simulink model "feedback_control"  (R2019a)
settings: Solver=FixedStepDiscrete  StartTime=0.0  StopTime=10.0  FixedStep=0.01  RelTol=1e-3
undefined symbols (not defined in the file): Adt, Bdt, c, DiscIntNeverNeededParam, pid, PID_pitch, PID_roll
libraries: simulink x2
settings Model: DataDictionary=pidSMC.sldd  Creator=david  LastModifiedBy=david

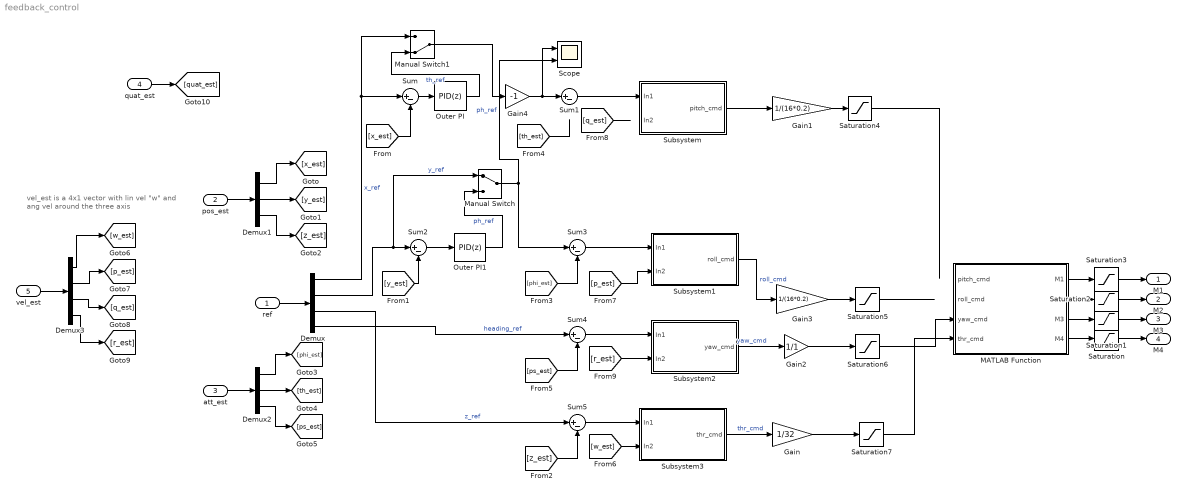
== system feedback_control ==
  note: vel_est is a 4x1 vector with lin vel "w" and
      | ang vel around the three axis
  ref : Inport
  pos_est : Inport  Port=2
  att_est : Inport  Port=3
  quat_est : Inport  Port=4
  vel_est : Inport  Port=5
  Demux : Demux
  Demux1 : Demux  Outputs=3
  Demux2 : Demux  Outputs=3
  Demux3 : Demux
  Gain : Gain  Gain=1/32
  Gain1 : Gain  Gain=1/(16*0.2)
  Gain2 : Gain  Gain=1/1
  Gain3 : Gain  Gain=1/(16*0.2)
  Gain4 : Gain  Gain=-1
  MATLAB Function : MATLAB Function  TreatAsAtomicUnit=on
  Manual Switch : ManualSwitch
  Manual Switch1 : ManualSwitch  CurrentSetting=0
  Outer PI : simulink/Continuous/PID Controller  Controller=PID  Form=Parallel  TimeDomain=Discrete-time  SampleTime=-1  IntegratorMethod=Forward Euler  FilterMethod=Forward Euler  ControllerParametersSource=internal  P=PID_pitch.Kp_out  I=PID_pitch.Ki_out  D=PID_pitch.Kd_out  UseFilter=off  N=pid.N  TunerSelectOption=Transfer Function Based (PID Tuner App)  InitialConditionSource=internal  InitialConditionForIntegrator=0  InitialConditionForFilter=0  DifferentiatorICPrevScaledInput=0  ExternalReset=none  TrackingMode=off  Kt=1  LimitOutput=on  UpperSaturationLimit=30/180*pi  LowerSaturationLimit=-30/180*pi  LinearizeAsGain=off  AntiWindupMode=clamping  Kb=1  POutMin=[]  POutMax=[]  IOutMin=[]  IOutMax=[]  DOutMin=[]  DOutMax=[]  NOutMin=[]  NOutMax=[]  SumOutMin=[]  SumOutMax=[]  SaturationOutMin=[]  SaturationOutMax=[]  PParamMin=[]  PParamMax=[]  IParamMin=[]  IParamMax=[]  DParamMin=[]  DParamMax=[]  NParamMin=[]  NParamMax=[]  KbParamMin=[]  KbParamMax=[]  KtParamMin=[]  KtParamMax=[]  KbOutMin=[]  KbOutMax=[]  KtOutMin=[]  KtOutMax=[]  IntegratorOutMin=[]  IntegratorOutMax=[]  FilterOutMin=[]  FilterOutMax=[]  SumI1OutMin=[]  SumI1OutMax=[]  SumI2OutMin=[]  SumI2OutMax=[]  SumI3OutMin=[]  SumI3OutMax=[]  SumI4OutMin=[]  SumI4OutMax=[]  SumDOutMin=[]  SumDOutMax=[]  DifferentiatorOutMin=[]  DifferentiatorOutMax=[]  FilterDiffOutCoefMin=[]  FilterDiffOutCoefMax=[]  ReciprocalOutMin=[]  ReciprocalOutMax=[]  SumDenOutMin=[]  SumDenOutMax=[]  SumNumOutMin=[]  SumNumOutMax=[]  DivideOutMin=[]  DivideOutMax=[]  IntegratorContinuousStateAttributes=''  IntegratorStateMustResolveToSignalObject=off  IntegratorRTWStateStorageClass=Auto  FilterContinuousStateAttributes=''  FilterStateMustResolveToSignalObject=off  FilterRTWStateStorageClass=Auto  ParallelPVariant=InternalParameters  IdealPVariant=Disabled  IVariant=InternalParameters  DVariant=InternalParameters  IntegratorVariant=Discrete  SatVariant=Enabled  AWVariant=DiscClampingParallel  PCopyVariant=Disabled  TRVariant=Disabled  FdbkBlocksVariant=Forward  IdealPFdbkVariant=Disabled  SatFdbkVariant=Disabled  DerivativeFilterVariant=Differentiator  NVariant=Passthrough  NCopyVariant=Disabled_SignalSpec  FilterICVariant=InternalICsDifferentiator  IntegratorICVariant=InternalICs  ExternalResetVariant=Disabled  TRSumVariant=Passthrough  SumFdbkVariant=Disabled  SumVariant=Sum_PID
  Outer PI1 : simulink/Continuous/PID Controller  Controller=PID  Form=Parallel  TimeDomain=Discrete-time  SampleTime=-1  IntegratorMethod=Forward Euler  FilterMethod=Forward Euler  ControllerParametersSource=internal  P=PID_roll.Kp_out  I=PID_roll.Ki_out  D=PID_roll.Kd_out  UseFilter=off  N=pid.N  TunerSelectOption=Transfer Function Based (PID Tuner App)  InitialConditionSource=internal  InitialConditionForIntegrator=0  InitialConditionForFilter=0  DifferentiatorICPrevScaledInput=0  ExternalReset=none  TrackingMode=off  Kt=1  LimitOutput=on  UpperSaturationLimit=30/180*pi  LowerSaturationLimit=-30/180*pi  LinearizeAsGain=off  AntiWindupMode=clamping  Kb=1  POutMin=[]  POutMax=[]  IOutMin=[]  IOutMax=[]  DOutMin=[]  DOutMax=[]  NOutMin=[]  NOutMax=[]  SumOutMin=[]  SumOutMax=[]  SaturationOutMin=[]  SaturationOutMax=[]  PParamMin=[]  PParamMax=[]  IParamMin=[]  IParamMax=[]  DParamMin=[]  DParamMax=[]  NParamMin=[]  NParamMax=[]  KbParamMin=[]  KbParamMax=[]  KtParamMin=[]  KtParamMax=[]  KbOutMin=[]  KbOutMax=[]  KtOutMin=[]  KtOutMax=[]  IntegratorOutMin=[]  IntegratorOutMax=[]  FilterOutMin=[]  FilterOutMax=[]  SumI1OutMin=[]  SumI1OutMax=[]  SumI2OutMin=[]  SumI2OutMax=[]  SumI3OutMin=[]  SumI3OutMax=[]  SumI4OutMin=[]  SumI4OutMax=[]  SumDOutMin=[]  SumDOutMax=[]  DifferentiatorOutMin=[]  DifferentiatorOutMax=[]  FilterDiffOutCoefMin=[]  FilterDiffOutCoefMax=[]  ReciprocalOutMin=[]  ReciprocalOutMax=[]  SumDenOutMin=[]  SumDenOutMax=[]  SumNumOutMin=[]  SumNumOutMax=[]  DivideOutMin=[]  DivideOutMax=[]  IntegratorContinuousStateAttributes=''  IntegratorStateMustResolveToSignalObject=off  IntegratorRTWStateStorageClass=Auto  FilterContinuousStateAttributes=''  FilterStateMustResolveToSignalObject=off  FilterRTWStateStorageClass=Auto  ParallelPVariant=InternalParameters  IdealPVariant=Disabled  IVariant=InternalParameters  DVariant=InternalParameters  IntegratorVariant=Discrete  SatVariant=Enabled  AWVariant=DiscClampingParallel  PCopyVariant=Disabled  TRVariant=Disabled  FdbkBlocksVariant=Forward  IdealPFdbkVariant=Disabled  SatFdbkVariant=Disabled  DerivativeFilterVariant=Differentiator  NVariant=Passthrough  NCopyVariant=Disabled_SignalSpec  FilterICVariant=InternalICsDifferentiator  IntegratorICVariant=InternalICs  ExternalResetVariant=Disabled  TRSumVariant=Passthrough  SumFdbkVariant=Disabled  SumVariant=Sum_PID
  Saturation : Saturate  UpperLimit=2000  LowerLimit=0
  Saturation1 : Saturate  UpperLimit=2000  LowerLimit=0
  Saturation2 : Saturate  UpperLimit=2000  LowerLimit=0
  Saturation3 : Saturate  UpperLimit=2000  LowerLimit=1000
  Saturation4 : Saturate  UpperLimit=1  LowerLimit=-1
  Saturation5 : Saturate  UpperLimit=1  LowerLimit=-1
  Saturation6 : Saturate  UpperLimit=1  LowerLimit=-1
  Saturation7 : Saturate  UpperLimit=1  LowerLimit=0
  Scope : Scope  NumInputPorts=2
  Subsystem : Subsystem
  Subsystem1 : Subsystem
  Subsystem2 : Subsystem
  Subsystem3 : Subsystem
  Sum{,1..5} (6 alike) : Sum  Inputs=|+-
  M1 : Outport
  M2 : Outport  Port=2
  M3 : Outport  Port=3
  M4 : Outport  Port=4
  wires:
  Outer PI/1 -> Manual Switch1/2  "th_ref"
  [x_est] -> Sum/2
  Saturation/1 -> M4/1
  Manual Switch/1 -> Sum3/1, Scope/2  "ph_ref"
  Demux/2 -> Manual Switch/1, Sum2/1  "y_ref"
  Gain3/1 -> Saturation5/1
  Gain/1 -> Saturation7/1
  Sum3/1 -> Subsystem1/1(In1)
  Outer PI1/1 -> Manual Switch/2  "ph_ref"
  ref/1 -> Demux/1
  Saturation2/1 -> M2/1
  vel_est/1 -> Demux3/1
  Demux3/1 -> [w_est]
  Gain1/1 -> Saturation4/1
  Saturation6/1 -> MATLAB Function/3(yaw_cmd)
  Gain2/1 -> Saturation6/1
  Gain4/1 -> Scope/1, Sum1/1
  Demux3/2 -> [p_est]
  MATLAB Function/2(M2) -> Saturation2/1
  Demux2/2 -> [th_est]
  Saturation3/1 -> M1/1
  [y_est] -> Sum2/2
  Saturation1/1 -> M3/1
  Saturation5/1 -> ?
  Demux3/3 -> [q_est]
  MATLAB Function/3(M3) -> Saturation1/1
  Saturation7/1 -> MATLAB Function/4(thr_cmd)
  Demux1/3 -> [z_est]
  Demux3/4 -> [r_est]
  Demux2/1 -> [phi_est]
  pos_est/1 -> Demux1/1
  Demux2/3 -> [ps_est]
  att_est/1 -> Demux2/1
  [phi_est] -> Sum3/2
  Demux1/2 -> [y_est]
  Demux1/1 -> [x_est]
  Demux/3 -> Sum5/1  "z_ref"
  [p_est] -> Subsystem1/2(In2)
  [r_est] -> Subsystem2/2(In2)
  Sum4/1 -> Subsystem2/1(In1)
  Subsystem1/1(roll_cmd) -> Gain3/1  "roll_cmd"
  [th_est] -> ?
  Subsystem2/1(yaw_cmd) -> Gain2/1  "yaw_cmd"
  Sum2/1 -> Outer PI1/1
  [ps_est] -> Sum4/2
  Demux/4 -> Sum4/1  "heading_ref"
  Subsystem3/1(thr_cmd) -> Gain/1  "thr_cmd"
  Sum/1 -> Outer PI/1
  Demux/1 -> Manual Switch1/1, Sum/1  "x_ref"
  MATLAB Function/1(M1) -> Saturation3/1
  [w_est] -> Subsystem3/2(In2)
  Saturation4/1 -> ?
  Sum5/1 -> Subsystem3/1(In1)
  Manual Switch1/1 -> Gain4/1
  [z_est] -> Sum5/2
  MATLAB Function/4(M4) -> Saturation/1
  Sum1/1 -> Subsystem/1(In1)
  [q_est] -> ?
  Subsystem/1(pitch_cmd) -> Gain1/1
  quat_est/1 -> [quat_est]

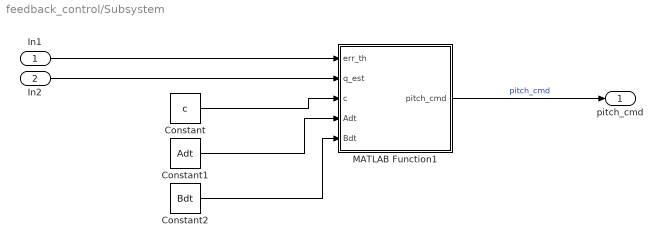
== system feedback_control/Subsystem ==
  In1 : Inport
  In2 : Inport  Port=2
  Constant : Constant  Value=c
  Constant1 : Constant  Value=Adt
  Constant2 : Constant  Value=Bdt
  MATLAB Function1 : MATLAB Function  TreatAsAtomicUnit=on
  pitch_cmd : Outport
  wires:
  MATLAB Function1/1(pitch_cmd) -> pitch_cmd/1  "pitch_cmd"
  In2/1 -> MATLAB Function1/2(q_est)
  In1/1 -> MATLAB Function1/1(err_th)
  Constant/1 -> MATLAB Function1/3(c)
  Constant1/1 -> MATLAB Function1/4(Adt)
  Constant2/1 -> MATLAB Function1/5(Bdt)

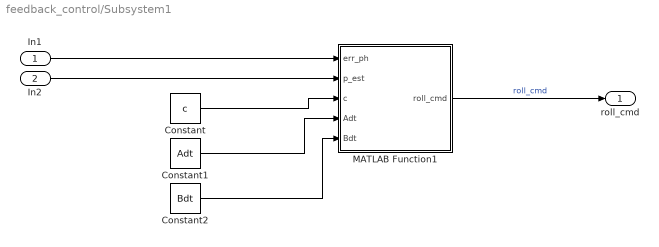
== system feedback_control/Subsystem1 ==
  In1 : Inport
  In2 : Inport  Port=2
  Constant : Constant  Value=c
  Constant1 : Constant  Value=Adt
  Constant2 : Constant  Value=Bdt
  MATLAB Function1 : MATLAB Function  TreatAsAtomicUnit=on
  roll_cmd : Outport
  wires:
  Constant2/1 -> MATLAB Function1/5(Bdt)
  Constant1/1 -> MATLAB Function1/4(Adt)
  Constant/1 -> MATLAB Function1/3(c)
  In1/1 -> MATLAB Function1/1(err_ph)
  In2/1 -> MATLAB Function1/2(p_est)
  MATLAB Function1/1(roll_cmd) -> roll_cmd/1  "roll_cmd"

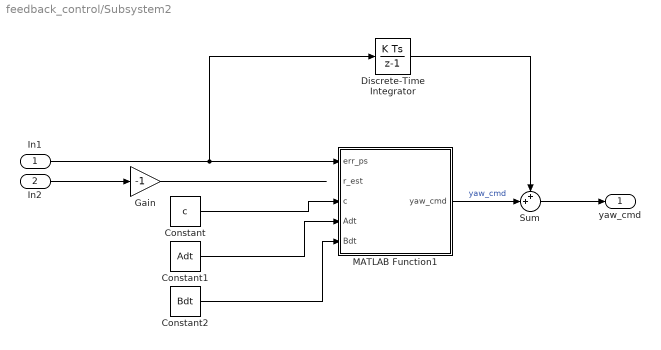
== system feedback_control/Subsystem2 ==
  In1 : Inport
  In2 : Inport  Port=2
  Constant : Constant  Value=c
  Constant1 : Constant  Value=Adt
  Constant2 : Constant  Value=Bdt
  Discrete-Time Integrator : DiscreteIntegrator  gainval=0.001  SampleTime=-1  ICPrevOutput=DiscIntNeverNeededParam  ICPrevScaledInput=DiscIntNeverNeededParam
  Gain : Gain  Gain=-1
  MATLAB Function1 : MATLAB Function  TreatAsAtomicUnit=on
  Sum : Sum  Inputs=++|
  yaw_cmd : Outport
  wires:
  MATLAB Function1/1(yaw_cmd) -> Sum/2  "yaw_cmd"
  In2/1 -> Gain/1
  In1/1 -> Discrete-Time Integrator/1, MATLAB Function1/1(err_ps)
  Constant/1 -> MATLAB Function1/3(c)
  Constant1/1 -> MATLAB Function1/4(Adt)
  Constant2/1 -> MATLAB Function1/5(Bdt)
  Sum/1 -> yaw_cmd/1
  Discrete-Time Integrator/1 -> Sum/1
  Gain/1 -> ?

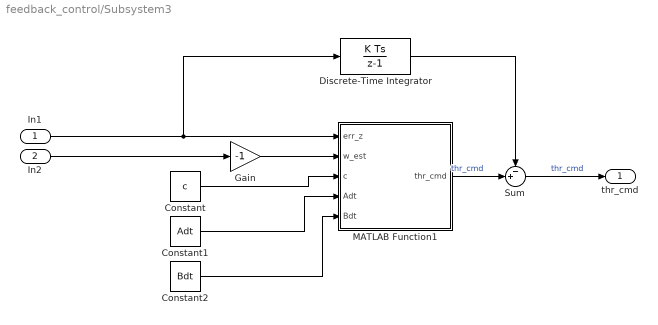
== system feedback_control/Subsystem3 ==
  In1 : Inport
  In2 : Inport  Port=2
  Constant : Constant  Value=c
  Constant1 : Constant  Value=Adt
  Constant2 : Constant  Value=Bdt
  Discrete-Time Integrator : DiscreteIntegrator  gainval=2  SampleTime=-1  LimitOutput=on  UpperSaturationLimit=20  LowerSaturationLimit=-20  ICPrevOutput=DiscIntNeverNeededParam  ICPrevScaledInput=DiscIntNeverNeededParam
  Gain : Gain  Gain=-1
  MATLAB Function1 : MATLAB Function  TreatAsAtomicUnit=on
  Sum : Sum  Inputs=-+|
  thr_cmd : Outport
  wires:
  Constant2/1 -> MATLAB Function1/5(Bdt)
  Constant1/1 -> MATLAB Function1/4(Adt)
  Constant/1 -> MATLAB Function1/3(c)
  Sum/1 -> thr_cmd/1  "thr_cmd"
  In2/1 -> Gain/1
  MATLAB Function1/1(thr_cmd) -> Sum/2  "thr_cmd"
  Discrete-Time Integrator/1 -> Sum/1
  Gain/1 -> MATLAB Function1/2(w_est)
  In1/1 -> MATLAB Function1/1(err_z), Discrete-Time Integrator/1

== matlab function feedback_control/Subsystem/MATLAB Function1 ==
  data: err_th input; pitch_cmd output; q_est input; c input; Adt input; Bdt input
function pitch_cmd = pitchSMC(err_th,q_est,c,Adt,Bdt)

pitch_cmd = inv(c'*Bdt)*c'*Adt*[ err_th; q_est ];

end

== matlab function feedback_control/MATLAB Function ==
  data: pitch_cmd input; M1 output; roll_cmd input; yaw_cmd input; thr_cmd input; M2 output; M3 output; M4 output
function [M1, M2, M3, M4] = motor_mixer(pitch_cmd, roll_cmd, yaw_cmd, thr_cmd)

idle = 1000;
K_thr = 800;
K_roll = 500;
K_pitch = 500;
K_yaw = 500;

% out = idle*ones(4,1) + K_thr*eye(4)*thr_cmd + K_roll*diag([-1, 1, 1, -1])*...
%     roll_cmd + K_pitch*diag([1, -1, 1, -1])*pitch_cmd + ...
%     K_yaw*diag([-1, -1, 1, 1])*yaw_cmd; % no matrix!

out = idle*ones(4,1) + K_thr*ones(4,1)*thr_cmd + K_roll*[-1, 1, 1, -1]'*...
    roll_cmd + K_pitch*[1, -1, 1, -1]'*pitch_cmd + ...
    K_yaw*[-1, -1, 1, 1]'*yaw_cmd; 



M1 = out(1);
M2 = out(2);
M3 = out(3);
M4 = out(4);
end

== matlab function feedback_control/Subsystem1/MATLAB Function1 ==
  data: err_ph input; roll_cmd output; p_est input; c input; Adt input; Bdt input
function roll_cmd = rollSMC(err_ph,p_est,c,Adt,Bdt)

roll_cmd = inv(c'*Bdt)*c'*Adt*[ err_ph; p_est ];

end

== matlab function feedback_control/Subsystem2/MATLAB Function1 ==
  data: err_ps input; yaw_cmd output; r_est input; c input; Adt input; Bdt input
function yaw_cmd = yawSMC(err_ps,r_est,c,Adt,Bdt)

c = [ 0.03; 1 ];
yaw_cmd = inv(c'*Bdt)*c'*Adt*[ err_ps; r_est ];

end

== matlab function feedback_control/Subsystem3/MATLAB Function1 ==
  data: err_z input; thr_cmd output; w_est input; c input; Adt input; Bdt input
function thr_cmd = thrustSMC(err_z,w_est,c,Adt,Bdt)

thr_cmd = -inv(c'*Bdt)*c'*Adt*[ err_z; w_est ];

end
